simulink model "maglev_model_2021"  (R2023b)
settings: Solver=VariableStepAuto  StartTime=0.0  StopTime=2  RelTol=1e-3
values from neighbouring files (symbols this model uses):
  g = 9.81    [planta_maglev.m]
  gamma = 328    [planta_maglev.m]
  i0 = 0.9487    [planta_maglev.m]
  k = 1.2E-4    (= 0.00012)    [planta_maglev.m]
  ki = 2*g / i0    (= 20.6809318014)    [planta_maglev.m]
  kx = -2*g / x0    (= -860.526315789)    [planta_maglev.m]
  m = 0.0212    [planta_maglev.m]
  rho = 0.166    [planta_maglev.m]
  x0 = 0.0228    [planta_maglev.m]
undefined symbols (not defined in the file or in its folder): magnitude
libraries: slpidlib x2
settings Model: Creator=aitor  LastModifiedBy=chris

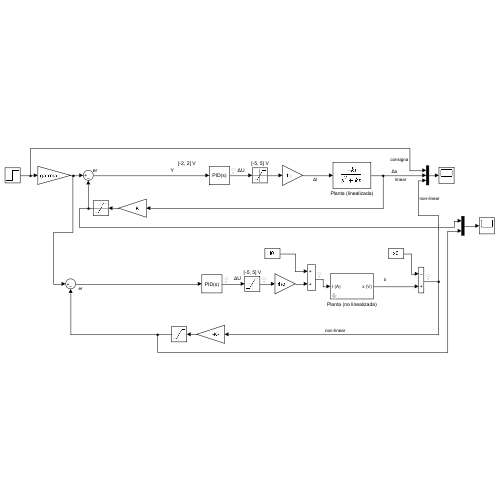
[thumbnail: Simulink's stored preview of the top-level diagram]
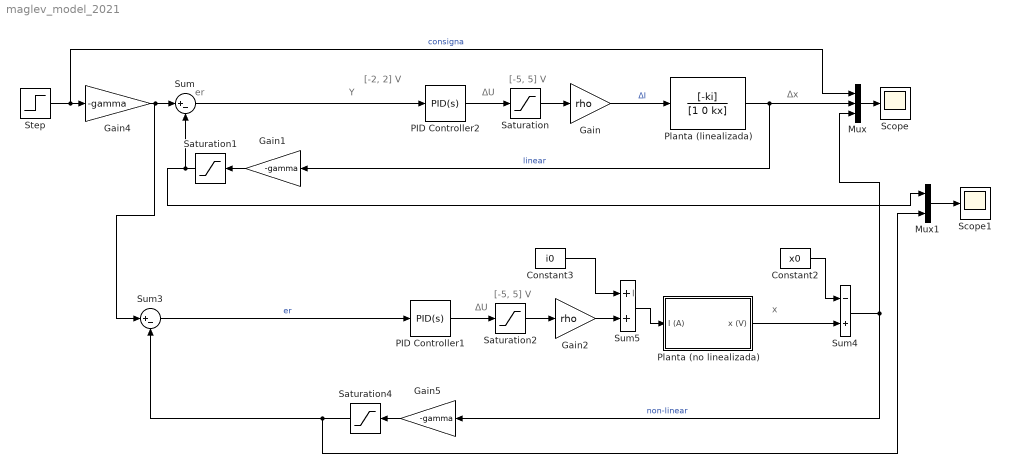
== system maglev_model_2021 ==
  note: [-2, 2] V
  note: Y
  note: er
  note: ΔU
  note: [-5, 5] V
  note: Δx
  note: I
  note: ΔU
  note: x
  note: [-5, 5] V
  Constant2 : Constant  Value=x0
  Constant3 : Constant  Value=i0
  Gain : Gain  Gain=rho
  Gain1 : Gain  Gain=-gamma
  Gain2 : Gain  Gain=rho
  Gain4 : Gain  Gain=-gamma
  Gain5 : Gain  Gain=-gamma
  Mux : Mux  Inputs=3
  Mux1 : Mux  Inputs=2
  PID Controller1 : slpidlib/PID Controller  Controller=PID  Form=Parallel  TimeDomain=Continuous-time  UseExternalTs=off  SampleTime=-1  IntegratorMethod=Forward Euler  FilterMethod=Forward Euler  ControllerParametersSource=internal  P=18.4157926253428  I=66.574639801784  UseKiTs=off  D=0.401108645856644  N=51667.197865857  UseFilter=on  TunerSelectOption=Transfer Function Based (PID Tuner App)  InitialConditionSource=internal  InitialConditionForIntegrator=0  InitialConditionForFilter=0  DifferentiatorICPrevScaledInput=0  ExternalReset=none  TrackingMode=off  Kt=1  LimitOutput=off  SatLimitsSource=internal  UpperSaturationLimit=5  LowerSaturationLimit=-5  LinearizeAsGain=on  AntiWindupMode=back-calculation  Kb=1  LimitIntegrator=off  UpperIntegratorSaturationLimit=inf  LowerIntegratorSaturationLimit=-inf  POutMin=[]  POutMax=[]  IOutMin=[]  IOutMax=[]  DOutMin=[]  DOutMax=[]  NOutMin=[]  NOutMax=[]  SumOutMin=[]  SumOutMax=[]  SaturationOutMin=[]  SaturationOutMax=[]  PParamMin=[]  PParamMax=[]  IParamMin=[]  IParamMax=[]  DParamMin=[]  DParamMax=[]  NParamMin=[]  NParamMax=[]  KbParamMin=[]  KbParamMax=[]  KtParamMin=[]  KtParamMax=[]  KbOutMin=[]  KbOutMax=[]  KtOutMin=[]  KtOutMax=[]  IntegratorOutMin=[]  IntegratorOutMax=[]  FilterOutMin=[]  FilterOutMax=[]  SumI1OutMin=[]  SumI1OutMax=[]  SumI2OutMin=[]  SumI2OutMax=[]  SumI3OutMin=[]  SumI3OutMax=[]  SumI4OutMin=[]  SumI4OutMax=[]  SumDOutMin=[]  SumDOutMax=[]  DifferentiatorOutMin=[]  DifferentiatorOutMax=[]  FilterDiffOutCoefMin=[]  FilterDiffOutCoefMax=[]  ReciprocalOutMin=[]  ReciprocalOutMax=[]  SumDenOutMin=[]  SumDenOutMax=[]  SumNumOutMin=[]  SumNumOutMax=[]  DivideOutMin=[]  DivideOutMax=[]  UdiffTsProdOutMin=[]  UdiffTsProdOutMax=[]  NTsProdOutMin=[]  NTsProdOutMax=[]  UintegralTsProdOutMin=[]  UintegralTsProdOutMax=[]  UngainTsProdOutMin=[]  UngainTsProdOutMax=[]  ClampingZeroOutDataTypeStr=Inherit: Inherit via back propagation  ClampingZeroOutMin=[]  ClampingZeroOutMax=[]  FilterDenConstantOutDataTypeStr=Inherit: Inherit via back propagation  FilterDenConstantOutMin=[]  FilterDenConstantOutMax=[]  PCopyOutDataTypeStr=Inherit: Inherit via back propagation  PCopyOutMin=[]  PCopyOutMax=[]  NCopyOutDataTypeStr=Inherit: Inherit via back propagation  NCopyOutMin=[]  NCopyOutMax=[]  IntegratorContinuousStateAttributes=''  IntegratorStateMustResolveToSignalObject=off  IntegratorRTWStateStorageClass=Auto  FilterContinuousStateAttributes=''  FilterStateMustResolveToSignalObject=off  FilterRTWStateStorageClass=Auto  ParallelPVariant=InternalParameters  IdealPVariant=Disabled  IVariant=InternalParameters  DVariant=InternalParameters  IntegratorVariant=Continuous  SatVariant=Disabled  AWVariant=Passthrough  PCopyVariant=Disabled  TRVariant=Disabled  FdbkBlocksVariant=Forward  IdealPFdbkVariant=Disabled  SatFdbkVariant=Disabled  DerivativeFilterVariant=ContFilter  NVariant=InternalParameters  NCopyVariant=Disabled  FilterICVariant=InternalICsFilter  IntegratorICVariant=InternalICs  ExternalResetVariant=Disabled  TRSumVariant=Passthrough  SumFdbkVariant=Disabled  SumVariant=Sum_PID  TsampFilterVariant=InternalTs  TsampNgainVariant=Passthrough  TsampIntegralVariant=Disabled_SignalSpec  ExternalSaturationOutDataTypeStr=Inherit: Same as second input
  PID Controller2 : slpidlib/PID Controller  Controller=PID  Form=Parallel  TimeDomain=Continuous-time  UseExternalTs=off  SampleTime=-1  IntegratorMethod=Forward Euler  FilterMethod=Forward Euler  ControllerParametersSource=internal  P=18.4157926253428  I=66.574639801784  UseKiTs=off  D=0.401108645856644  N=51667.197865857  UseFilter=on  TunerSelectOption=Transfer Function Based (PID Tuner App)  InitialConditionSource=internal  InitialConditionForIntegrator=0  InitialConditionForFilter=0  DifferentiatorICPrevScaledInput=0  ExternalReset=none  TrackingMode=off  Kt=1  LimitOutput=off  SatLimitsSource=internal  UpperSaturationLimit=5  LowerSaturationLimit=-5  LinearizeAsGain=on  AntiWindupMode=back-calculation  Kb=1  LimitIntegrator=off  UpperIntegratorSaturationLimit=inf  LowerIntegratorSaturationLimit=-inf  POutMin=[]  POutMax=[]  IOutMin=[]  IOutMax=[]  DOutMin=[]  DOutMax=[]  NOutMin=[]  NOutMax=[]  SumOutMin=[]  SumOutMax=[]  SaturationOutMin=[]  SaturationOutMax=[]  PParamMin=[]  PParamMax=[]  IParamMin=[]  IParamMax=[]  DParamMin=[]  DParamMax=[]  NParamMin=[]  NParamMax=[]  KbParamMin=[]  KbParamMax=[]  KtParamMin=[]  KtParamMax=[]  KbOutMin=[]  KbOutMax=[]  KtOutMin=[]  KtOutMax=[]  IntegratorOutMin=[]  IntegratorOutMax=[]  FilterOutMin=[]  FilterOutMax=[]  SumI1OutMin=[]  SumI1OutMax=[]  SumI2OutMin=[]  SumI2OutMax=[]  SumI3OutMin=[]  SumI3OutMax=[]  SumI4OutMin=[]  SumI4OutMax=[]  SumDOutMin=[]  SumDOutMax=[]  DifferentiatorOutMin=[]  DifferentiatorOutMax=[]  FilterDiffOutCoefMin=[]  FilterDiffOutCoefMax=[]  ReciprocalOutMin=[]  ReciprocalOutMax=[]  SumDenOutMin=[]  SumDenOutMax=[]  SumNumOutMin=[]  SumNumOutMax=[]  DivideOutMin=[]  DivideOutMax=[]  UdiffTsProdOutMin=[]  UdiffTsProdOutMax=[]  NTsProdOutMin=[]  NTsProdOutMax=[]  UintegralTsProdOutMin=[]  UintegralTsProdOutMax=[]  UngainTsProdOutMin=[]  UngainTsProdOutMax=[]  ClampingZeroOutDataTypeStr=Inherit: Inherit via back propagation  ClampingZeroOutMin=[]  ClampingZeroOutMax=[]  FilterDenConstantOutDataTypeStr=Inherit: Inherit via back propagation  FilterDenConstantOutMin=[]  FilterDenConstantOutMax=[]  PCopyOutDataTypeStr=Inherit: Inherit via back propagation  PCopyOutMin=[]  PCopyOutMax=[]  NCopyOutDataTypeStr=Inherit: Inherit via back propagation  NCopyOutMin=[]  NCopyOutMax=[]  IntegratorContinuousStateAttributes=''  IntegratorStateMustResolveToSignalObject=off  IntegratorRTWStateStorageClass=Auto  FilterContinuousStateAttributes=''  FilterStateMustResolveToSignalObject=off  FilterRTWStateStorageClass=Auto  ParallelPVariant=InternalParameters  IdealPVariant=Disabled  IVariant=InternalParameters  DVariant=InternalParameters  IntegratorVariant=Continuous  SatVariant=Disabled  AWVariant=Passthrough  PCopyVariant=Disabled  TRVariant=Disabled  FdbkBlocksVariant=Forward  IdealPFdbkVariant=Disabled  SatFdbkVariant=Disabled  DerivativeFilterVariant=ContFilter  NVariant=InternalParameters  NCopyVariant=Disabled  FilterICVariant=InternalICsFilter  IntegratorICVariant=InternalICs  ExternalResetVariant=Disabled  TRSumVariant=Passthrough  SumFdbkVariant=Disabled  SumVariant=Sum_PID  TsampFilterVariant=InternalTs  TsampNgainVariant=Passthrough  TsampIntegralVariant=Disabled_SignalSpec  ExternalSaturationOutDataTypeStr=Inherit: Same as second input
  Planta (linealizada) : TransferFcn  Numerator=[-ki]  Denominator=[1 0 kx]
  Planta (no linealizada) : Subsystem  mask{k=k, m=m, g=g}
  Saturation : Saturate  UpperLimit=5  LowerLimit=-5
  Saturation1 : Saturate  UpperLimit=2  LowerLimit=-2
  Saturation2 : Saturate  UpperLimit=5  LowerLimit=-5
  Saturation4 : Saturate  UpperLimit=2  LowerLimit=-2
  Scope : Scope
  Scope1 : Scope
  Step : Step  Before=-0.005  After=0.004  SampleTime=0
  Sum : Sum  Inputs=|+-
  Sum3 : Sum  Inputs=|+-
  Sum4 : Sum  Inputs=-+
  Sum5 : Sum
  wires:
  Planta (linealizada)/1 -> Gain1/1, Mux/2  "linear"
  Saturation/1 -> Gain/1
  Sum/1 -> PID Controller2/1
  Mux/1 -> Scope/1
  PID Controller2/1 -> Saturation/1
  Constant3/1 -> Sum5/1
  Sum5/1 -> Planta (no linealizada)/1(I (A))
  PID Controller1/1 -> Saturation2/1
  Gain2/1 -> Sum5/2
  Step/1 -> Gain4/1, Mux/1  "consigna"
  Saturation2/1 -> Gain2/1
  Planta (no linealizada)/1(x (V)) -> Sum4/2
  Gain/1 -> Planta (linealizada)/1  "ΔI"
  Sum4/1 -> Gain5/1, Mux/3  "non-linear"
  Constant2/1 -> Sum4/1
  Mux1/1 -> Scope1/1
  Gain1/1 -> Saturation1/1
  Saturation1/1 -> Mux1/1, Sum/2
  Gain4/1 -> Sum3/1, Sum/1
  Gain5/1 -> Saturation4/1
  Saturation4/1 -> Mux1/2, Sum3/2
  Sum3/1 -> PID Controller1/1  "er"

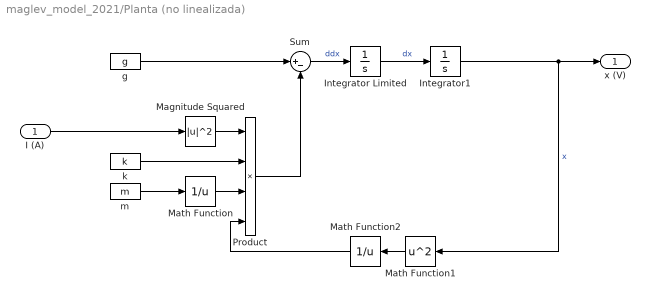
== system maglev_model_2021/Planta (no linealizada) ==
  I (A) : Inport
  Integrator Limited : Integrator  UpperSaturationLimit=100  LowerSaturationLimit=-100
  Integrator1 : Integrator  InitialCondition=0.0227  LimitOutput=on  LowerSaturationLimit=0.01
  Magnitude Squared : Math  Operator=magnitude^2
  Math Function : Math  Operator=reciprocal  OutputSignalType=real
  Math Function1 : Math  Operator=square  OutputSignalType=real  OutMin=[0.1]  OutDataTypeStr=double
  Math Function2 : Math  Operator=reciprocal  OutputSignalType=real
  Product : Product  Inputs=4
  Sum : Sum  Inputs=|+-
  g : Constant  Value=g
  k : Constant  Value=k
  m : Constant  Value=m
  x (V) : Outport
  wires:
  Sum/1 -> Integrator Limited/1  "ddx"
  Integrator Limited/1 -> Integrator1/1  "dx"
  Integrator1/1 -> Math Function1/1, x (V)/1  "x"
  g/1 -> Sum/1
  I (A)/1 -> Magnitude Squared/1
  m/1 -> Math Function/1
  Magnitude Squared/1 -> Product/1
  k/1 -> Product/2
  Math Function/1 -> Product/3
  Product/1 -> Sum/2
  Math Function1/1 -> Math Function2/1
  Math Function2/1 -> Product/4
